simulink model "window_in_stream_out_rtp"  (R2019b)
settings: Solver=VariableStepAuto  StartTime=0.0  StopTime=7  RelTol=1e-3
undefined symbols (not defined in the file): xc7vx485tffg1157
libraries: ModelComposer x5
settings Model: Creator=viswanad  LastModifiedBy=abehbood
settings DataIOCC: ReturnWorkspaceOutputs=off
settings SFSimCC: CustomCodeUndefinedFunction=UseInterfaceOnly

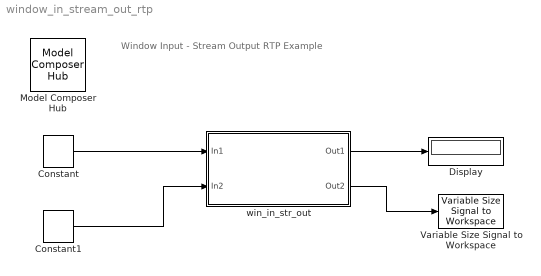
== system window_in_stream_out_rtp ==
  note: Window Input - Stream Output RTP Example
  Constant : ModelComposer/Constant  Value=[1 2 3 4 5 6 7 8 1 2 3 4 5 6 7 8]  SampleTime=1  OutDataType=int16  TypeExp=''  Signedness=Signed  WordLength=16  FractionalLength=0  RoundingMode=Truncation to minus infinity  OverflowMode=Wrap around
  Constant1 : ModelComposer/Constant  Value=[1 2 3 4]  SampleTime=1  OutDataType=int8  TypeExp=''  Signedness=Signed  WordLength=16  FractionalLength=0  RoundingMode=Truncation to minus infinity  OverflowMode=Wrap around
  Display : Display
  Model Composer Hub : ModelComposer/Model Composer Hub  CodeGeneration=off  SubsystemName=win_in_str_out  TargetDirectory=./code_async  ExportType=AI Engines  IpVendor=xilinx.com  IpLibrary=hls  IpVersion=1.0  IpHWLanguage=Verilog  AieCompilerOptions={}  CreateTestbench=on  TestbenchStackSize=10  RunAieSim=on  AieSimTimeout=50000  LaunchVitisAnalyzer=off  RunX86Sim=off  X86SimTimeout=10  ProjDevice=xc7vx485tffg1157-1  ProjDevicePart=xc7vx485tffg1157-1  SamplePeriod=-1  ClockFrequency=200  DataPathParallelism=1
  Variable Size Signal to Workspace : ModelComposer/Variable Size Signal to Workspace  VariableNameMask=simout
  win_in_str_out : Subsystem
  wires:
  Constant/1 -> win_in_str_out/1(In1)
  win_in_str_out/1(Out1) -> Display/1
  win_in_str_out/2(Out2) -> Variable Size Signal to Workspace/1
  Constant1/1 -> win_in_str_out/2(In2)

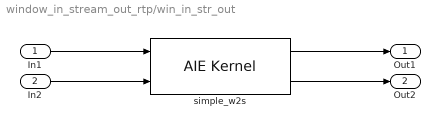
== system window_in_stream_out_rtp/win_in_str_out ==
  In1 : Inport
  In2 : Inport  Port=2
  simple_w2s : ModelComposer/AIE Kernel  PortAttributesTable={ 'Input', 'in1', 'input_window_int16 *', '16', '0', 'sync', ''; 'Inout', 'io_rtp', 'int8 &', '', '', 'async', '1'; 'Input', 'coeff', 'int8 const ( &) [ 4 ]', '', '', 'async', '4'; 'Output', 'out', 'output_stream_int32 *', '', '', '', '16' }  PortAttributesEnablement={'off', 'off', 'off', 'on', 'on', 'on', 'off';'off', 'off', 'off', 'off', 'off', 'on', 'off';'off', 'off', 'off', 'off', 'off', 'on', 'off';'off', 'off', 'off', 'off', 'off', 'off', 'on'}  FormalArgDecls={'input_window_int16 * in1', 'int8 & io_rtp', 'int8 const ( & coeff ) [ 4 ]', 'output_stream_int32 * out'}  PortWindowSizes={1.600000000000000000e+01; 0.000000000000000000e+00; 0.000000000000000000e+00; 0.000000000000000000e+00}  PortWindowMargins={0.000000000000000000e+00; 0.000000000000000000e+00; 0.000000000000000000e+00; 0.000000000000000000e+00}  PortSynchronicities={'sync'; 'async'; 'async'; 'auto'}  PortSignalSizes={0.000000000000000000e+00; 1.000000000000000000e+00; 4.000000000000000000e+00; 1.600000000000000000e+01}  SimLibPath=''  FunctionTabVisible=on  FunctionDescription=void simple_w2s(input_window_int16 * in1, int8 & io_rtp, int8 const ( & coeff ) [ 4 ], output_stream_int32 * out)  KernelHeaderFile=src/kernels/window_in_stream_out_rtp.h  KernelFunction=simple_w2s  KernelFunctionSelect=<empty>  KernelSourceFile=src/kernels/window_in_stream_out_rtp.cc  KernelSearchPaths={}  PreProcOptions={}  CoreRuntimeRatio=0.9  KernelLocSpec=off  ColRowLocation=[0 0]
  Out1 : Outport  VectorParamsAs1DForOutWhenUnconnected=off
  Out2 : Outport  Port=2  VectorParamsAs1DForOutWhenUnconnected=off
  wires:
  In1/1 -> simple_w2s/1
  simple_w2s/1 -> Out1/1
  simple_w2s/2 -> Out2/1
  In2/1 -> simple_w2s/2
